simulink model "Task10"  (R2019b)
settings: Solver=VariableStepAuto  StartTime=0.0  StopTime=10.0  RelTol=1e-3
settings Model: Creator=12393  LastModifiedBy=12393

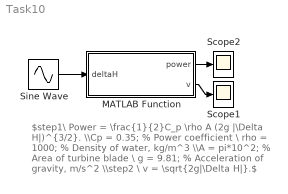
== system Task10 ==
  note: $step1\ Power = \frac{1}{2}C_p \rho A (2g |\Delta H|)^{3/2}. \\Cp = 0.35; % Power coefficient \ rho = 1000; % Density of water, kg/m^3 \\A = pi*10^2; % Area of turbine blade \ g = 9.81; % Acceleration of gravity, m/s^2 \\step2 \ v = \sqrt{2g|\Delta H|}.$
  MATLAB Function : MATLAB Function  TreatAsAtomicUnit=on
  Scope1 : Scope
  Scope2 : Scope
  Sine Wave : Sin  Amplitude=0.75  Frequency=0.5  SampleTime=0
  wires:
  MATLAB Function/2(v) -> Scope1/1
  Sine Wave/1 -> MATLAB Function/1(deltaH)
  MATLAB Function/1(power) -> Scope2/1

== matlab function Task10/MATLAB Function ==
  data: deltaH input; power output; v output
function [power,v]= fcn(deltaH)

Cp = 0.35; % Power coefficient
rho = 1000; % Density of water, kg/m^3
A = pi*10^2; % Area of turbine blade
g = 9.81; % Acceleration of gravity, m/s^2

power =0.5*Cp*rho*A*(2*g*abs(deltaH))^(3/2);
v=sqrt(2*g*abs(deltaH));
